simulink model "Eigenvalue"  (R2019b)
settings: Solver=VariableStepAuto  StartTime=0.0  StopTime=10.0  RelTol=1e-3
values from neighbouring files (symbols this model uses):
  A = zeros(4,4)    [Code.m]    (also in matlab.mat = [0 -2.58 0 0.08 1 0 0 0 0 0.08 0 -0.08 ... (16 elements, 4x4)
  B = [0 0 0 1/J]'    [Code.m]    (also in matlab.mat = [0 0 0 1])
  C = eye(4)    [Code.m]    (also in matlab.mat = [1 0 0 0 0 1 0 0 0 0 1 0 ... (16 elements, 4x4)])
  D = zeros(4,1)    [Code.m]    (also in matlab.mat = [0 0 0 0])
  Delta_X_Initial_Conditions = X_Initial_Conditions - Xss    [Code.m]    (also in matlab.mat = [-0.0523598775598 0.095 -2.75868926439 0.095])
  F = place(A,B,lambda_desired)    [Code.m]    (also in matlab.mat = [79587.5162501 40579.25 534.36 38])
settings Model: Creator=keeyanhaghshenas  LastModifiedBy=keeyanhaghshenas

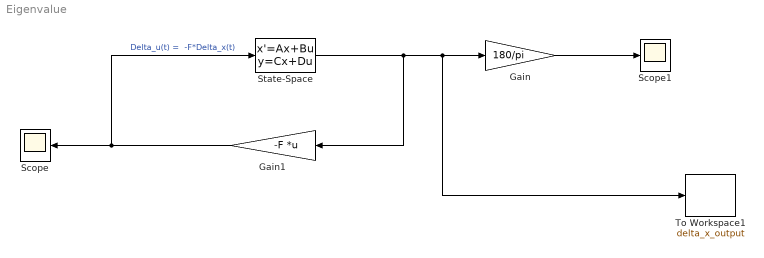
== system Eigenvalue ==
  Gain : Gain  Gain=180/pi
  Gain1 : Gain  Gain=-F  Multiplication=Matrix(K*u)
  Scope : Scope
  Scope1 : Scope
  State-Space : StateSpace  A=A  B=B  C=C  D=D  InitialCondition=Delta_X_Initial_Conditions
  To Workspace1 : ToWorkspace  VariableName=delta_x_output  SampleTime=-1
      settings: Save2DSignal=2-D array (concatenate along first dimension)
  wires:
  Gain/1 -> Scope1/1
  Gain1/1 -> State-Space/1, Scope/1  "Delta_u(t) =  -F*Delta_x(t)"
  State-Space/1 -> Gain1/1, To Workspace1/1, Gain/1
